simulink model "generate_joint_velocity_motion"  (R2025a)
settings: Solver=FixedStepDiscrete  StartTime=0.0  StopTime=inf  FixedStep=0.001  RelTol=1e-3
PreLoadFcn:
  | frs = FrankaRobotSettings;
libraries: franka_simulink x1
settings Model: SimulationMode=external  ExtModeTrigDuration=10000  Creator=vasi_ko  LastModifiedBy=kvasios
settings SolverCC: ConcurrentTasks=on  AlgebraicLoopSolver=TrustRegion
settings DataIOCC: LimitDataPoints=on  SaveFormat=Array  ReturnWorkspaceOutputs=off
settings OptimizationCC: EnhancedBackFolding=on  PassReuseOutputArgsThreshold=0.0  MaxStackSize=64  OptimizeBlockOrder=speed  DifferentSizesBufferReuse=on  OptimizationCustomize=off
settings DebuggingCC: SolverPrmCheckMsg=warning  ParameterTunabilityLossMsg=error  UnconnectedInputMsg=warning  UnconnectedOutputMsg=warning  UnconnectedLineMsg=warning  SFUnexpectedBacktrackingDiag=warning  SFNoUnconditionalDefaultTransitionDiag=warning  SFExecutionAtInitializationDiag=none  ArithmeticOperatorsInVariantConditions=warning
settings HardwareCC: ProdBitPerLong=64.0  ProdHWDeviceType=Intel->x86-64 (Linux 64)
settings ModelReferenceCC: EnableRefExpFcnMdlSchedulingChecks=on  PropagateSignalLabelsOutOfModel=off
settings SFSimCC: SimUseLocalCustomCode=off  MATLABDynamicMemAlloc=off  CustomCodeUndefinedFunction=UseInterfaceOnly  SimTargetLang=C++  SimDLTargetLibrary=mkl-dnn
settings RTWCC: HardwareBoard=Generic Linux AMD64 Board  RTWVerbose=off  RTWUseLocalCustomCode=off  BuildConfiguration=Faster Runs  TargetLang=C++  GPUComputeCapability=3.5  DLArmComputeVersion=19.05
settings CodeAppCC: ForceParamTrailComments=on  OperatorAnnotations=on
settings GRTTargetCC: ExtModeStaticAlloc=on  ExtModeMexFile=ext_xcp  ExtModeIntrfLevel=Level2 - Open
settings ConfigComp: CovMetricSettings=dw  CovSaveCumulativeToWorkspaceVar=on  CovSaveSingleToWorkspaceVar=on  CovExternalEMLEnable=off  CovSFcnEnable=off

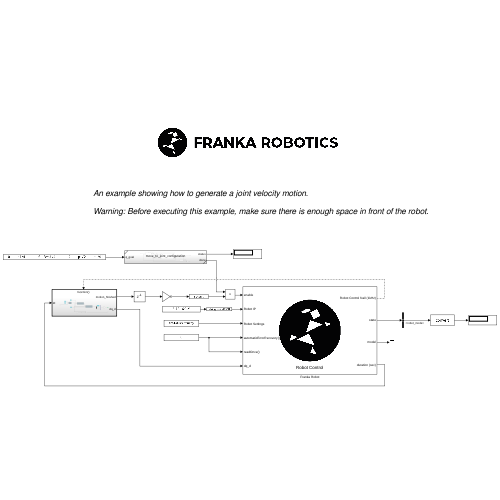
[thumbnail: Simulink's stored preview of the top-level diagram]
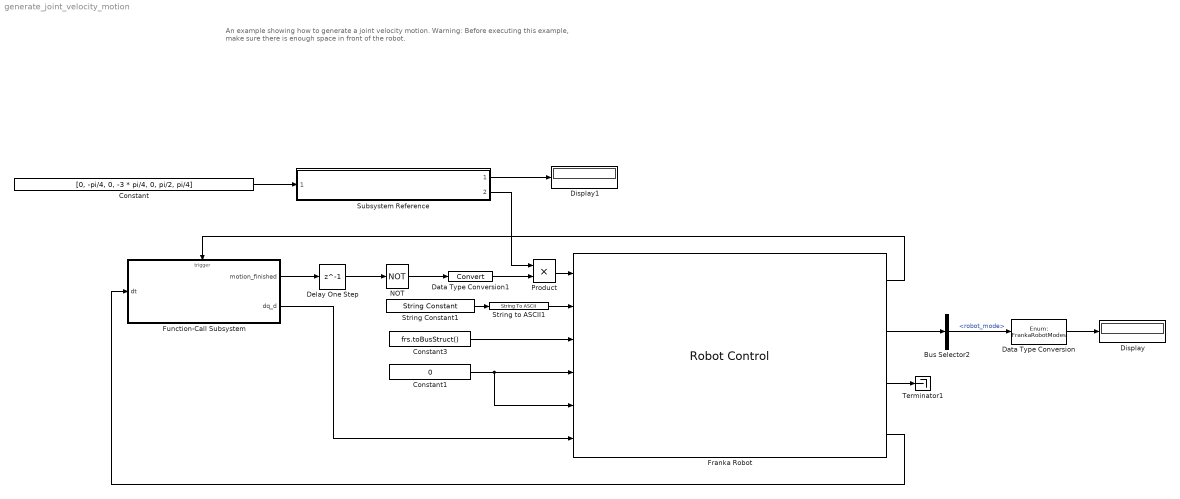
== system generate_joint_velocity_motion ==
  note: An example showing how to generate a joint velocity motion.
      |
      | Warning: Before executing this example, make sure there is enough space in front of the robot.
  Bus Selector2 : BusSelector  OutputSignals=robot_mode
  Constant : Constant  Value=[0, -pi/4, 0, -3 * pi/4, 0, pi/2, pi/4]
  Constant1 : Constant  Value=0  OutDataTypeStr=Bus: FrankaRobotSettingsBus
  Constant3 : Constant  Value=frs.toBusStruct()  OutDataTypeStr=Bus: FrankaRobotSettingsBus
  Data Type Conversion : DataTypeConversion  OutDataTypeStr=Enum: FrankaRobotModes  SaturateOnIntegerOverflow=off  RndMeth=Floor
  Data Type Conversion1 : DataTypeConversion  SaturateOnIntegerOverflow=off  RndMeth=Floor
  Delay One Step : Delay  DelayLength=1
  Display : Display
  Display1 : Display
  Franka Robot : franka_simulink/Robot Control  control_mode=Joint Velocities
      settings: SourceProductName=Franka Robotics Simulink Support Package
  Function-Call Subsystem : Subsystem  TreatAsAtomicUnit=on
      settings: RTWSystemCode=Nonreusable function
  NOT : Logic  Operator=NOT  IconShape=distinctive  AllPortsSameDT=off  OutDataTypeStr=boolean
  Product : Product
  String Constant1 : StringConstant  String="\"172.16.0.2\""
  String to ASCII1 : StringToASCII  OutputVectorSize=16
  Subsystem Reference : Subsystem  ReferencedSubsystem=move_to_joint_configuration
  Terminator1 : Terminator
  wires:
  Data Type Conversion/1 -> Display/1
  Franka Robot/2 -> Bus Selector2/1
  Function-Call Subsystem/1(motion_finished) -> Delay One Step/1
  Franka Robot/3 -> Terminator1/1
  Function-Call Subsystem/2(dq_d) -> Franka Robot/6
  Franka Robot/4 -> Function-Call Subsystem/1(dt)
  Delay One Step/1 -> NOT/1
  Franka Robot/1 -> Function-Call Subsystem/Trigger
  String Constant1/1 -> String to ASCII1/1
  Bus Selector2/1 -> Data Type Conversion/1  "<robot_mode>"
  Constant3/1 -> Franka Robot/3
  String to ASCII1/1 -> Franka Robot/2
  NOT/1 -> Data Type Conversion1/1
  Subsystem Reference/2 -> Product/1
  Constant/1 -> Subsystem Reference/1
  Product/1 -> Franka Robot/1
  Data Type Conversion1/1 -> Product/2
  Constant1/1 -> Franka Robot/5, Franka Robot/4
  Subsystem Reference/1 -> Display1/1

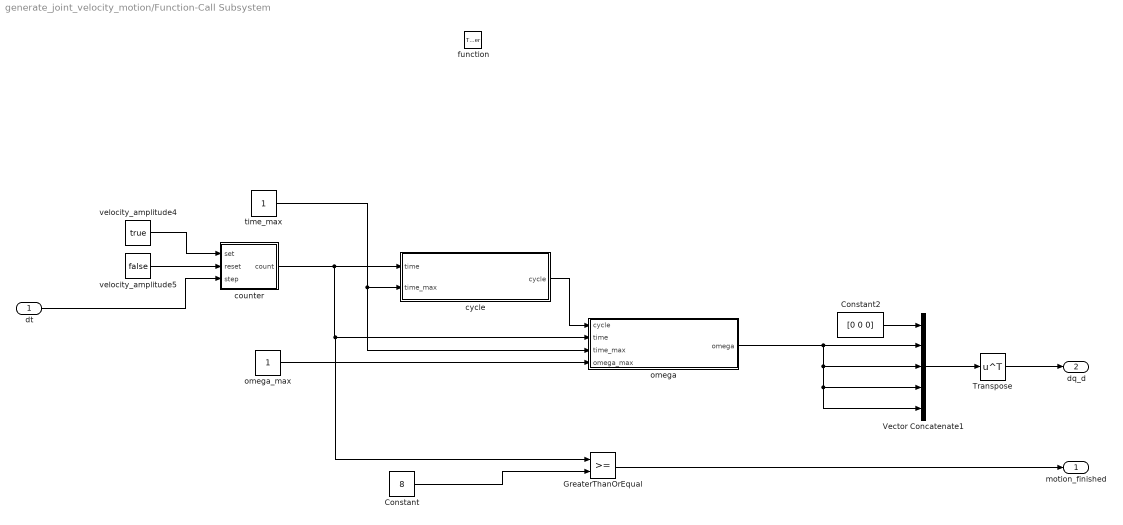
== system generate_joint_velocity_motion/Function-Call Subsystem ==
  dt : Inport
  function : TriggerPort  TriggerType=function-call  VariantControl=(inherit)
  Constant : Constant  Value=8
  Constant2 : Constant  Value=[0 0 0]  VectorParams1D=off
  GreaterThanOrEqual : RelationalOperator  OutDataTypeStr=boolean  RndMeth=Simplest  InputSameDT=off
  Transpose : Math  Operator=transpose
  Vector Concatenate1 : Concatenate  NumInputs=5
  counter : Subsystem
  cycle : Subsystem
  omega : Subsystem
  omega_max : Constant  VectorParams1D=off
  time_max : Constant  VectorParams1D=off
  velocity_amplitude4 : Constant  Value=true  VectorParams1D=off
  velocity_amplitude5 : Constant  Value=false  VectorParams1D=off
  motion_finished : Outport  InitialOutput=0
  dq_d : Outport  Port=2  VectorParamsAs1DForOutWhenUnconnected=off
  wires:
  omega/1(omega) -> Vector Concatenate1/5, Vector Concatenate1/4, Vector Concatenate1/3, Vector Concatenate1/2
  Vector Concatenate1/1 -> Transpose/1
  cycle/1(cycle) -> omega/1(cycle)
  counter/1(count) -> cycle/1(time), GreaterThanOrEqual/1, omega/2(time)
  omega_max/1 -> omega/4(omega_max)
  Constant2/1 -> Vector Concatenate1/1
  Transpose/1 -> dq_d/1
  time_max/1 -> omega/3(time_max), cycle/2(time_max)
  velocity_amplitude5/1 -> counter/2(reset)
  velocity_amplitude4/1 -> counter/1(set)
  dt/1 -> counter/3(step)
  Constant/1 -> GreaterThanOrEqual/2
  GreaterThanOrEqual/1 -> motion_finished/1

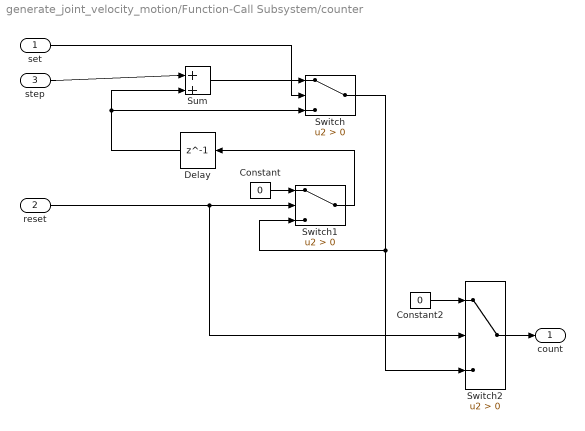
== system generate_joint_velocity_motion/Function-Call Subsystem/counter ==
  set : Inport  OutDataTypeStr=boolean
  reset : Inport  Port=2  OutDataTypeStr=boolean
  step : Inport  Port=3  OutDataTypeStr=double
  Constant : Constant  Value=0  OutDataTypeStr=double
  Constant2 : Constant  Value=0  OutDataTypeStr=double
  Delay : Delay  DelayLength=1  InitialCondition=0
  Sum : Sum  Inputs=|++
  Switch : Switch  Criteria=u2 > Threshold  SaturateOnIntegerOverflow=off  InputSameDT=off
  Switch1 : Switch  Criteria=u2 > Threshold  OutDataTypeStr=double  SaturateOnIntegerOverflow=off  InputSameDT=off
  Switch2 : Switch  Criteria=u2 > Threshold  OutDataTypeStr=double  SaturateOnIntegerOverflow=off  InputSameDT=off
  count : Outport  OutDataTypeStr=double  VectorParamsAs1DForOutWhenUnconnected=off
  wires:
  Switch2/1 -> count/1
  Constant2/1 -> Switch2/1
  Sum/1 -> Switch/1
  set/1 -> Switch/2
  Switch/1 -> Switch1/3, Switch2/3
  step/1 -> Sum/1
  Delay/1 -> Sum/2, Switch/3
  reset/1 -> Switch1/2, Switch2/2
  Constant/1 -> Switch1/1
  Switch1/1 -> Delay/1

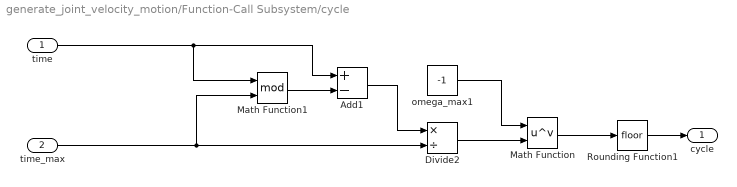
== system generate_joint_velocity_motion/Function-Call Subsystem/cycle ==
  time : Inport
  time_max : Inport  Port=2
  Add1 : Sum  Inputs=+-
  Divide2 : Product  Inputs=*/
  Math Function : Math  Operator=pow  SignedPower=on
  Math Function1 : Math  Operator=mod  SignedPower=on
  Rounding Function1 : Rounding
  omega_max1 : Constant  Value=-1  VectorParams1D=off
  cycle : Outport  InitialOutput=[0 0 0 0 0 0 0]  VectorParamsAs1DForOutWhenUnconnected=off
  wires:
  Divide2/1 -> Math Function/2
  Math Function1/1 -> Add1/2
  time/1 -> Add1/1, Math Function1/1
  time_max/1 -> Math Function1/2, Divide2/2
  Rounding Function1/1 -> cycle/1
  Math Function/1 -> Rounding Function1/1
  omega_max1/1 -> Math Function/1
  Add1/1 -> Divide2/1

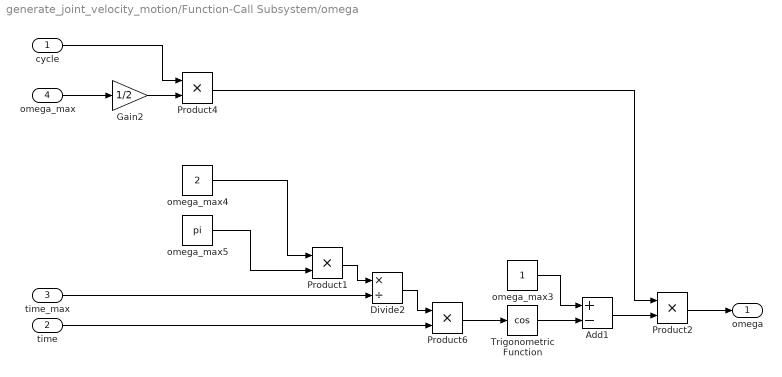
== system generate_joint_velocity_motion/Function-Call Subsystem/omega ==
  cycle : Inport
  time : Inport  Port=2
  time_max : Inport  Port=3
  omega_max : Inport  Port=4
  Add1 : Sum  Inputs=+-
  Divide2 : Product  Inputs=*/
  Gain2 : Gain  Gain=1/2
  Product{1..2,4,6} (4 alike) : Product
  Trigonometric Function : Trigonometry  Operator=cos
  omega_max3 : Constant  VectorParams1D=off
  omega_max4 : Constant  Value=2  VectorParams1D=off
  omega_max5 : Constant  Value=pi  VectorParams1D=off
  omega : Outport  InitialOutput=[0 0 0 0 0 0 0]  VectorParamsAs1DForOutWhenUnconnected=off
  wires:
  cycle/1 -> Product4/1
  omega_max/1 -> Gain2/1
  Product4/1 -> Product2/1
  Gain2/1 -> Product4/2
  omega_max3/1 -> Add1/1
  omega_max5/1 -> Product1/2
  omega_max4/1 -> Product1/1
  Divide2/1 -> Product6/1
  Product1/1 -> Divide2/1
  Product6/1 -> Trigonometric Function/1
  Trigonometric Function/1 -> Add1/2
  time_max/1 -> Divide2/2
  time/1 -> Product6/2
  Add1/1 -> Product2/2
  Product2/1 -> omega/1
